simulink model "benchmarkss"  (Simulink 10.0)
settings: Solver=ode15s  StartTime=0.0  StopTime=200  FixedStep=0.01  RelTol=1e-5  AbsTol=1e-8
undefined symbols (not defined in the file or in its folder): carb1, carb2, carb3, carb4, carb5, carb6, carb7, KLa1, KLa2, KLa3, KLa4, KLa5, KLa6, KLa7, metal1, metal2, metal3, metal4, metal5, metal6, metal7, Qin0, Qintr, Qw
settings Model: Creator=ielulf  LastModifiedBy=xfal  ExtModeTrigMode=oneshot  ExtModeArmWhenConnect=off  ExtModeAutoUpdateStatusClock=off
settings SolverCC: AutoScaleAbsTol=off
settings DataIOCC: SignalLoggingSaveFormat=ModelDataLogs  SaveOutput=off  TimeSaveName=t  SignalLoggingName=sigsOut  OutputTimes=[0:(1):150]
settings OptimizationCC: BlockReduction=off  BooleanDataType=off  ExpressionDepthLimit=2147483647  InitFltsAndDblsToZero=on
settings DebuggingCC: AlgebraicLoopMsg=none  SaveWithParameterizedLinksMsg=none  SignalResolutionControl=TryResolveAllWithWarning  InheritedTsInSrcMsg=none  MultiTaskDSMMsg=warning  MultiTaskCondExecSysMsg=none  FcnCallInpInsideContextMsg=warning  UnconnectedOutputMsg=none  StateNameClashWarn=warning
settings HardwareCC: TargetUnknown=on
settings SFSimCC: SimUseLocalCustomCode=on  CustomCodeUndefinedFunction=FilterOut
settings RTWCC: TemplateMakefile=grt_unix.tmf  RTWUseLocalCustomCode=on
settings GRTTargetCC: TargetFcnLib=ansi_tfl_tmw.mat

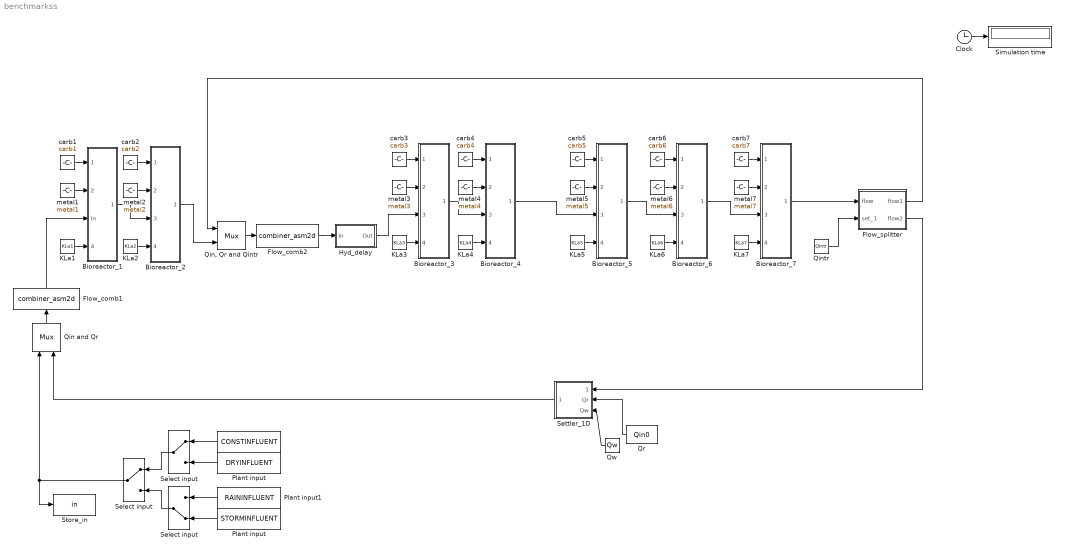
== system benchmarkss ==
  " " : FromWorkspace  VariableName=CONSTINFLUENT  OutputAfterFinalValue=Holding final value
  " Select input" : ManualSwitch
  Bioreactor_1 : Subsystem
  Bioreactor_2 : Subsystem
  Bioreactor_3 : Subsystem
  Bioreactor_4 : Subsystem
  Bioreactor_5 : Subsystem
  Bioreactor_6 : Subsystem
  Bioreactor_7 : Subsystem
  Clock : Clock
  Flow_comb1 : S-Function  FunctionName=combiner_asm2d  SFunctionDeploymentMode=off  EnableBusSupport=off
  Flow_comb2 : S-Function  FunctionName=combiner_asm2d  SFunctionDeploymentMode=off  EnableBusSupport=off
  Flow_splitter : Subsystem
  Hyd_delay : Subsystem
  KLa1 : Constant  Value=KLa1
  KLa2 : Constant  Value=KLa2
  KLa3 : Constant  Value=KLa3
  KLa4 : Constant  Value=KLa4
  KLa5 : Constant  Value=KLa5
  KLa6 : Constant  Value=KLa6
  KLa7 : Constant  Value=KLa7
  Plant input : FromWorkspace  VariableName=DRYINFLUENT  OutputAfterFinalValue=Holding final value
  "Plant input " : FromWorkspace  VariableName=STORMINFLUENT  OutputAfterFinalValue=Holding final value
  Plant input1 : FromWorkspace  VariableName=RAININFLUENT  OutputAfterFinalValue=Holding final value
  Qin and Qr : Mux  Inputs=2
  "Qin, Qr and Qintr" : Mux  Inputs=2
  Qintr : Constant  Value=Qintr
  Qr : Constant  Value=Qin0
  Qw : Constant  Value=Qw
  Select input : ManualSwitch
  "Select input " : ManualSwitch  CurrentSetting=0
  Settler_1D : Subsystem
  Simulation time : Display
  Store_in : ToWorkspace  VariableName=in  SampleTime=-1
  carb1 : Constant  Value=carb1
  carb2 : Constant  Value=carb2
  carb3 : Constant  Value=carb3
  carb4 : Constant  Value=carb4
  carb5 : Constant  Value=carb5
  carb6 : Constant  Value=carb6
  carb7 : Constant  Value=carb7
  metal1 : Constant  Value=metal1
  metal2 : Constant  Value=metal2
  metal3 : Constant  Value=metal3
  metal4 : Constant  Value=metal4
  metal5 : Constant  Value=metal5
  metal6 : Constant  Value=metal6
  metal7 : Constant  Value=metal7
  wires:
  Clock/1 -> Simulation time/1
  carb1/1 -> Bioreactor_1/1(carb)
  KLa1/1 -> Bioreactor_1/4(KLa)
  metal1/1 -> Bioreactor_1/2(metal)
  Flow_comb1/1 -> Bioreactor_1/3(in)
  Qin and Qr/1 -> Flow_comb1/1
  Plant input/1 -> Select input/2
  " "/1 -> Select input/1
  Plant input1/1 -> "Select input "/1
  "Plant input "/1 -> "Select input "/2
  Select input/1 -> " Select input"/1
  "Select input "/1 -> " Select input"/2
  " Select input"/1 -> Store_in/1, Qin and Qr/1
  Settler_1D/1(output) -> Qin and Qr/2
  Qw/1 -> Settler_1D/3(Qw)
  Qr/1 -> Settler_1D/2(Qr)
  Flow_splitter/2(flow2) -> Settler_1D/1(feed)
  "Qin, Qr and Qintr"/1 -> Flow_comb2/1
  Flow_comb2/1 -> Hyd_delay/1(In)
  KLa2/1 -> Bioreactor_2/4(KLa2)
  carb2/1 -> Bioreactor_2/1(carb2)
  metal2/1 -> Bioreactor_2/2(metal2)
  Bioreactor_1/1(out) -> Bioreactor_2/3(in1)
  Bioreactor_2/1(out1) -> "Qin, Qr and Qintr"/2
  KLa3/1 -> Bioreactor_3/4(KLa3)
  carb3/1 -> Bioreactor_3/1(carb3)
  metal3/1 -> Bioreactor_3/2(metal3)
  Hyd_delay/1(Out) -> Bioreactor_3/3(in1)
  KLa4/1 -> Bioreactor_4/4(KLa4)
  carb4/1 -> Bioreactor_4/1(carb4)
  metal4/1 -> Bioreactor_4/2(metal4)
  Bioreactor_3/1(out1) -> Bioreactor_4/3(in1)
  KLa5/1 -> Bioreactor_5/4(KLa5)
  carb5/1 -> Bioreactor_5/1(carb5)
  metal5/1 -> Bioreactor_5/2(metal5)
  Bioreactor_4/1(out1) -> Bioreactor_5/3(in1)
  KLa6/1 -> Bioreactor_6/4(KLa6)
  carb6/1 -> Bioreactor_6/1(carb6)
  metal6/1 -> Bioreactor_6/2(metal6)
  Bioreactor_5/1(out1) -> Bioreactor_6/3(in1)
  KLa7/1 -> Bioreactor_7/4(KLa7)
  carb7/1 -> Bioreactor_7/1(carb7)
  metal7/1 -> Bioreactor_7/2(metal7)
  Bioreactor_6/1(out1) -> Bioreactor_7/3(in1)
  Qintr/1 -> Flow_splitter/2(set_1)
  Bioreactor_7/1(out1) -> Flow_splitter/1(flow)
  Flow_splitter/1(flow1) -> "Qin, Qr and Qintr"/1

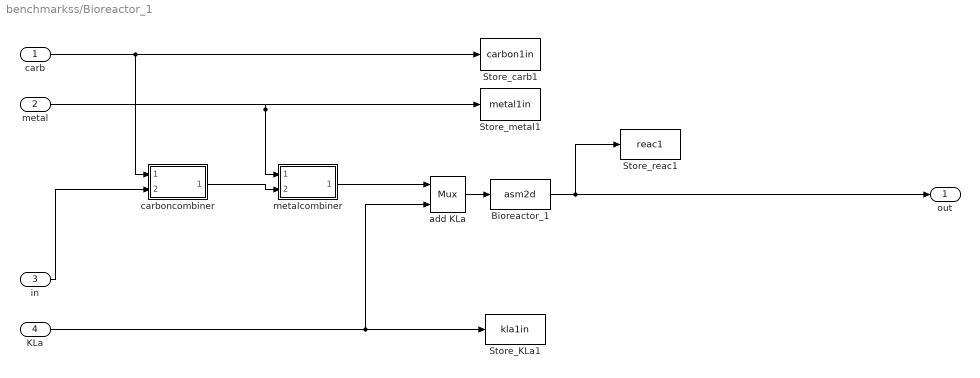
== system benchmarkss/Bioreactor_1 ==
  carb : Inport
  metal : Inport  Port=2
  in : Inport  Port=3
  KLa : Inport  Port=4
  Bioreactor_1 : S-Function  FunctionName=asm2d  Parameters=XINIT1,PAR1,VOL1,SOSAT1, DECAY, TEMPMODEL, ACTIVATE  SFunctionDeploymentMode=off  EnableBusSupport=off
  Store_KLa1 : ToWorkspace  VariableName=kla1in  SampleTime=-1
  Store_carb1 : ToWorkspace  VariableName=carbon1in  SampleTime=-1
  Store_metal1 : ToWorkspace  VariableName=metal1in  SampleTime=-1
  Store_reac1 : ToWorkspace  VariableName=reac1  SampleTime=-1
  add KLa : Mux  Inputs=2
  carboncombiner : Subsystem
  metalcombiner : Subsystem
  out : Outport
  wires:
  Bioreactor_1/1 -> Store_reac1/1, out/1
  in/1 -> carboncombiner/2(Input)
  KLa/1 -> Store_KLa1/1, add KLa/2
  carboncombiner/1(Output) -> metalcombiner/2(Input)
  metal/1 -> metalcombiner/1(C_flow), Store_metal1/1
  metalcombiner/1(Output) -> add KLa/1
  carb/1 -> carboncombiner/1(C_flow), Store_carb1/1
  add KLa/1 -> Bioreactor_1/1

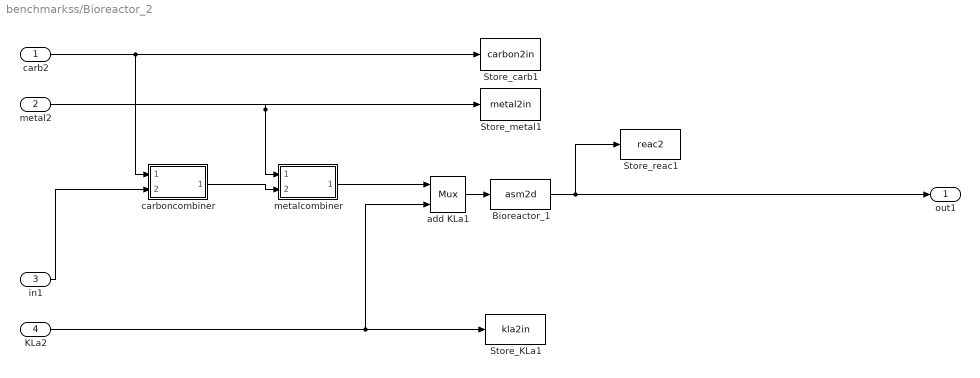
== system benchmarkss/Bioreactor_2 ==
  carb2 : Inport
  metal2 : Inport  Port=2
  in1 : Inport  Port=3
  KLa2 : Inport  Port=4
  Bioreactor_1 : S-Function  FunctionName=asm2d  Parameters=XINIT2,PAR2,VOL2,SOSAT2, DECAY, TEMPMODEL, ACTIVATE  SFunctionDeploymentMode=off  EnableBusSupport=off
  Store_KLa1 : ToWorkspace  VariableName=kla2in  SampleTime=-1
  Store_carb1 : ToWorkspace  VariableName=carbon2in  SampleTime=-1
  Store_metal1 : ToWorkspace  VariableName=metal2in  SampleTime=-1
  Store_reac1 : ToWorkspace  VariableName=reac2  SampleTime=-1
  add KLa1 : Mux  Inputs=2
  carboncombiner : Subsystem
  metalcombiner : Subsystem
  out1 : Outport
  wires:
  add KLa1/1 -> Bioreactor_1/1
  Bioreactor_1/1 -> Store_reac1/1, out1/1
  in1/1 -> carboncombiner/2(Input)
  KLa2/1 -> Store_KLa1/1, add KLa1/2
  carboncombiner/1(Output) -> metalcombiner/2(Input)
  metal2/1 -> metalcombiner/1(C_flow), Store_metal1/1
  metalcombiner/1(Output) -> add KLa1/1
  carb2/1 -> carboncombiner/1(C_flow), Store_carb1/1

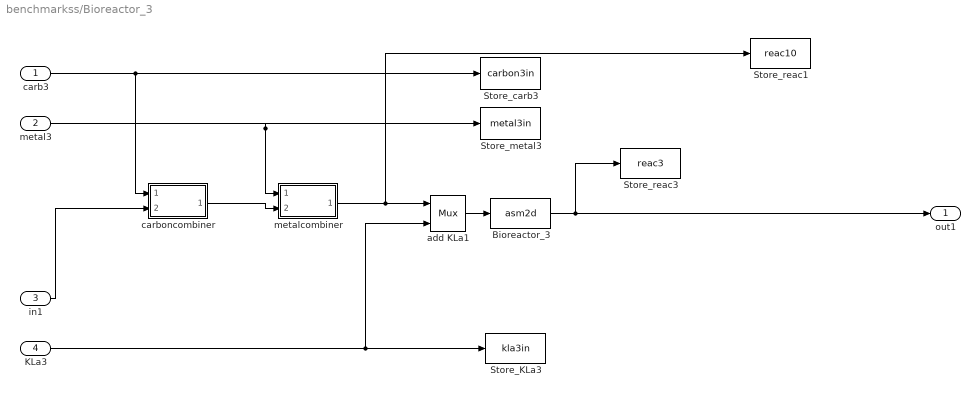
== system benchmarkss/Bioreactor_3 ==
  carb3 : Inport
  metal3 : Inport  Port=2
  in1 : Inport  Port=3
  KLa3 : Inport  Port=4
  Bioreactor_3 : S-Function  FunctionName=asm2d  Parameters=XINIT3,PAR3,VOL3,SOSAT3, DECAY,TEMPMODEL, ACTIVATE  SFunctionDeploymentMode=off  EnableBusSupport=off
  Store_KLa3 : ToWorkspace  VariableName=kla3in  SampleTime=-1
  Store_carb3 : ToWorkspace  VariableName=carbon3in  SampleTime=-1
  Store_metal3 : ToWorkspace  VariableName=metal3in  SampleTime=-1
  Store_reac1 : ToWorkspace  VariableName=reac10  SampleTime=-1
  Store_reac3 : ToWorkspace  VariableName=reac3  SampleTime=-1
  add KLa1 : Mux  Inputs=2
  carboncombiner : Subsystem
  metalcombiner : Subsystem
  out1 : Outport
  wires:
  add KLa1/1 -> Bioreactor_3/1
  Bioreactor_3/1 -> Store_reac3/1, out1/1
  in1/1 -> carboncombiner/2(Input)
  KLa3/1 -> Store_KLa3/1, add KLa1/2
  carboncombiner/1(Output) -> metalcombiner/2(Input)
  metal3/1 -> metalcombiner/1(C_flow), Store_metal3/1
  metalcombiner/1(Output) -> add KLa1/1, Store_reac1/1
  carb3/1 -> carboncombiner/1(C_flow), Store_carb3/1

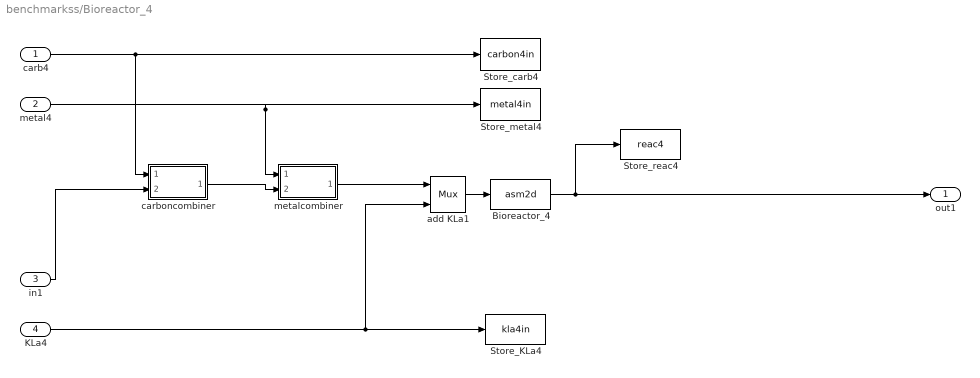
== system benchmarkss/Bioreactor_4 ==
  carb4 : Inport
  metal4 : Inport  Port=2
  in1 : Inport  Port=3
  KLa4 : Inport  Port=4
  Bioreactor_4 : S-Function  FunctionName=asm2d  Parameters=XINIT4,PAR4,VOL4,SOSAT4, DECAY,TEMPMODEL, ACTIVATE  SFunctionDeploymentMode=off  EnableBusSupport=off
  Store_KLa4 : ToWorkspace  VariableName=kla4in  SampleTime=-1
  Store_carb4 : ToWorkspace  VariableName=carbon4in  SampleTime=-1
  Store_metal4 : ToWorkspace  VariableName=metal4in  SampleTime=-1
  Store_reac4 : ToWorkspace  VariableName=reac4  SampleTime=-1
  add KLa1 : Mux  Inputs=2
  carboncombiner : Subsystem
  metalcombiner : Subsystem
  out1 : Outport
  wires:
  add KLa1/1 -> Bioreactor_4/1
  Bioreactor_4/1 -> Store_reac4/1, out1/1
  in1/1 -> carboncombiner/2(Input)
  KLa4/1 -> Store_KLa4/1, add KLa1/2
  carboncombiner/1(Output) -> metalcombiner/2(Input)
  metal4/1 -> metalcombiner/1(C_flow), Store_metal4/1
  metalcombiner/1(Output) -> add KLa1/1
  carb4/1 -> carboncombiner/1(C_flow), Store_carb4/1

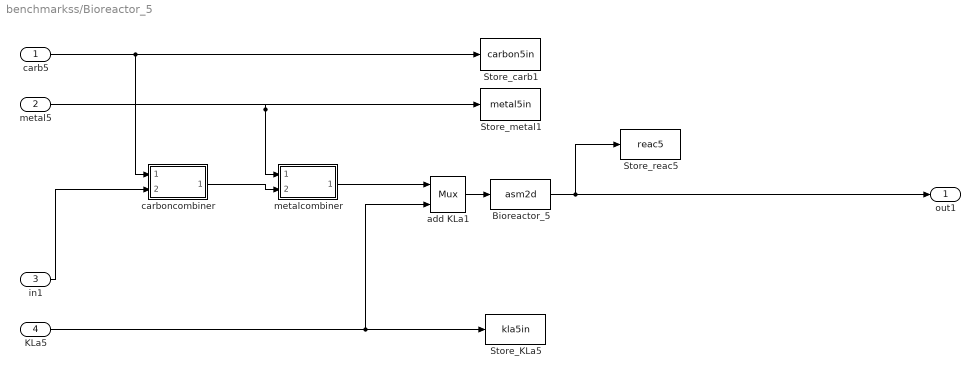
== system benchmarkss/Bioreactor_5 ==
  carb5 : Inport
  metal5 : Inport  Port=2
  in1 : Inport  Port=3
  KLa5 : Inport  Port=4
  Bioreactor_5 : S-Function  FunctionName=asm2d  Parameters=XINIT5,PAR5,VOL5,SOSAT5, DECAY, TEMPMODEL, ACTIVATE  SFunctionDeploymentMode=off  EnableBusSupport=off
  Store_KLa5 : ToWorkspace  VariableName=kla5in  SampleTime=-1
  Store_carb1 : ToWorkspace  VariableName=carbon5in  SampleTime=-1
  Store_metal1 : ToWorkspace  VariableName=metal5in  SampleTime=-1
  Store_reac5 : ToWorkspace  VariableName=reac5  SampleTime=-1
  add KLa1 : Mux  Inputs=2
  carboncombiner : Subsystem
  metalcombiner : Subsystem
  out1 : Outport
  wires:
  add KLa1/1 -> Bioreactor_5/1
  Bioreactor_5/1 -> Store_reac5/1, out1/1
  in1/1 -> carboncombiner/2(Input)
  KLa5/1 -> Store_KLa5/1, add KLa1/2
  carboncombiner/1(Output) -> metalcombiner/2(Input)
  metal5/1 -> metalcombiner/1(C_flow), Store_metal1/1
  metalcombiner/1(Output) -> add KLa1/1
  carb5/1 -> carboncombiner/1(C_flow), Store_carb1/1

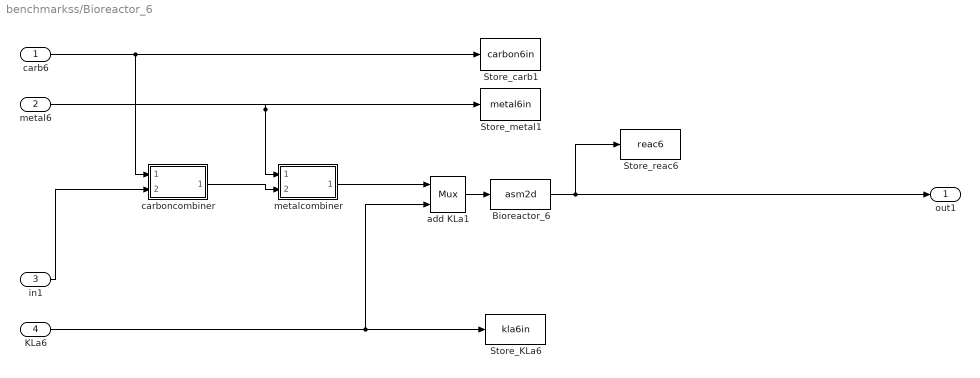
== system benchmarkss/Bioreactor_6 ==
  carb6 : Inport
  metal6 : Inport  Port=2
  in1 : Inport  Port=3
  KLa6 : Inport  Port=4
  Bioreactor_6 : S-Function  FunctionName=asm2d  Parameters=XINIT6,PAR6,VOL6,SOSAT6, DECAY, TEMPMODEL, ACTIVATE  SFunctionDeploymentMode=off  EnableBusSupport=off
  Store_KLa6 : ToWorkspace  VariableName=kla6in  SampleTime=-1
  Store_carb1 : ToWorkspace  VariableName=carbon6in  SampleTime=-1
  Store_metal1 : ToWorkspace  VariableName=metal6in  SampleTime=-1
  Store_reac6 : ToWorkspace  VariableName=reac6  SampleTime=-1
  add KLa1 : Mux  Inputs=2
  carboncombiner : Subsystem
  metalcombiner : Subsystem
  out1 : Outport
  wires:
  add KLa1/1 -> Bioreactor_6/1
  Bioreactor_6/1 -> Store_reac6/1, out1/1
  in1/1 -> carboncombiner/2(Input)
  KLa6/1 -> Store_KLa6/1, add KLa1/2
  carboncombiner/1(Output) -> metalcombiner/2(Input)
  metal6/1 -> metalcombiner/1(C_flow), Store_metal1/1
  metalcombiner/1(Output) -> add KLa1/1
  carb6/1 -> carboncombiner/1(C_flow), Store_carb1/1

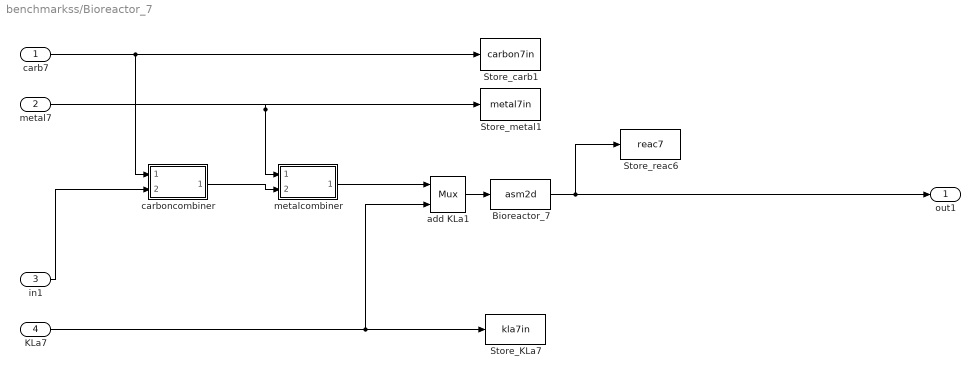
== system benchmarkss/Bioreactor_7 ==
  carb7 : Inport
  metal7 : Inport  Port=2
  in1 : Inport  Port=3
  KLa7 : Inport  Port=4
  Bioreactor_7 : S-Function  FunctionName=asm2d  Parameters=XINIT7,PAR7,VOL7,SOSAT7, DECAY, TEMPMODEL, ACTIVATE  SFunctionDeploymentMode=off  EnableBusSupport=off
  Store_KLa7 : ToWorkspace  VariableName=kla7in  SampleTime=-1
  Store_carb1 : ToWorkspace  VariableName=carbon7in  SampleTime=-1
  Store_metal1 : ToWorkspace  VariableName=metal7in  SampleTime=-1
  Store_reac6 : ToWorkspace  VariableName=reac7  SampleTime=-1
  add KLa1 : Mux  Inputs=2
  carboncombiner : Subsystem
  metalcombiner : Subsystem
  out1 : Outport
  wires:
  add KLa1/1 -> Bioreactor_7/1
  Bioreactor_7/1 -> Store_reac6/1, out1/1
  in1/1 -> carboncombiner/2(Input)
  KLa7/1 -> Store_KLa7/1, add KLa1/2
  carboncombiner/1(Output) -> metalcombiner/2(Input)
  metal7/1 -> metalcombiner/1(C_flow), Store_metal1/1
  metalcombiner/1(Output) -> add KLa1/1
  carb7/1 -> carboncombiner/1(C_flow), Store_carb1/1

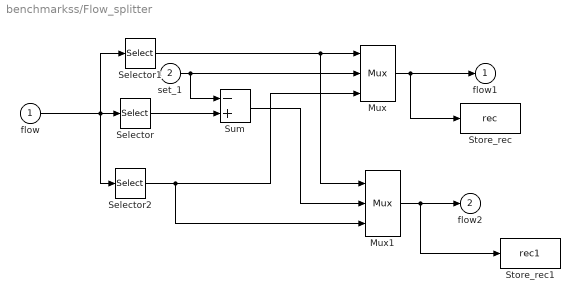
== system benchmarkss/Flow_splitter ==
  flow : Inport
  set_1 : Inport  Port=2
  Mux : Mux  Inputs=3
  Mux1 : Mux  Inputs=3
  Selector : Selector  InputPortWidth=26  IndexOptions=Index vector (dialog)  Indices=[20]  OutputSizes=1
  Selector1 : Selector  InputPortWidth=26  IndexOptions=Index vector (dialog)  Indices=[1 2 3 4 5 6 7 8 9 10 11 12 13 14 15 16 17 18 19 ]  OutputSizes=1
  Selector2 : Selector  InputPortWidth=26  IndexOptions=Index vector (dialog)  Indices=[21 22 23 24 25 26]  OutputSizes=1
  Store_rec : ToWorkspace  VariableName=rec  SampleTime=-1
  Store_rec1 : ToWorkspace  VariableName=rec1  SampleTime=-1
  Sum : Sum  Inputs=-+  SaturateOnIntegerOverflow=on  InputSameDT=on  OutDataTypeStr=Inherit: Same as first input
  flow1 : Outport
  flow2 : Outport  Port=2
  wires:
  flow/1 -> Selector1/1, Selector/1, Selector2/1
  Mux/1 -> flow1/1, Store_rec/1
  Mux1/1 -> flow2/1, Store_rec1/1
  set_1/1 -> Mux/2, Sum/1
  Selector/1 -> Sum/2
  Sum/1 -> Mux1/2
  Selector1/1 -> Mux/1, Mux1/1
  Selector2/1 -> Mux/3, Mux1/3

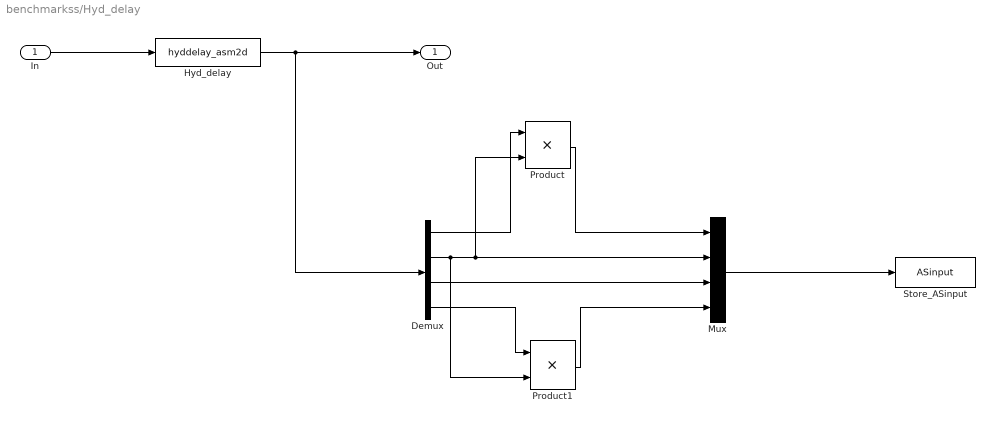
== system benchmarkss/Hyd_delay ==
  In : Inport
  Demux : Demux  Outputs=[19,1,1,5]
  Hyd_delay : S-Function  FunctionName=hyddelay_asm2d  Parameters=XINITDELAY,PAR1, T  SFunctionDeploymentMode=off  EnableBusSupport=off
  Mux : Mux
  Product : Product  SaturateOnIntegerOverflow=on  OutDataTypeStr=Inherit: Same as first input
  Product1 : Product  SaturateOnIntegerOverflow=on  OutDataTypeStr=Inherit: Same as first input
  Store_ASinput : ToWorkspace  VariableName=ASinput  SampleTime=-1
  Out : Outport
  wires:
  In/1 -> Hyd_delay/1
  Hyd_delay/1 -> Out/1, Demux/1
  Demux/1 -> Product/1
  Product/1 -> Mux/1
  Mux/1 -> Store_ASinput/1
  Demux/4 -> Product1/1
  Product1/1 -> Mux/4
  Demux/3 -> Mux/3
  Demux/2 -> Product1/2, Mux/2, Product/2

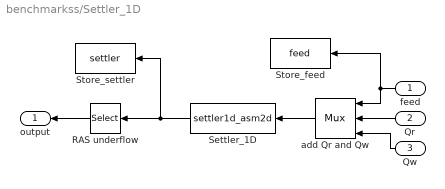
== system benchmarkss/Settler_1D ==
  feed : Inport
  Qr : Inport  Port=2
  Qw : Inport  Port=3
  RAS underflow : Selector  InputPortWidth=316  IndexOptions=Index vector (dialog)  Indices=[1 2 3 4 5 6 7 8 9 10 11 12 13 14 15 16 17 18 19 20 21 22 23 24 25 26]  OutputSizes=1
  Settler_1D : S-Function  FunctionName=settler1d_asm2d  Parameters=SETTLERINIT2D,SETTLERPAR2D,DIM2D,LAYER2D,ASM2DPAR, DECAY, SETTLER, TEMPMODEL  SFunctionDeploymentMode=off  EnableBusSupport=off
  Store_feed : ToWorkspace  VariableName=feed  SampleTime=-1
  Store_settler : ToWorkspace  VariableName=settler  SampleTime=-1
  add Qr and Qw : Mux  Inputs=3
  output : Outport
  wires:
  add Qr and Qw/1 -> Settler_1D/1
  Qr/1 -> add Qr and Qw/2
  Qw/1 -> add Qr and Qw/3
  feed/1 -> add Qr and Qw/1, Store_feed/1
  RAS underflow/1 -> output/1
  Settler_1D/1 -> RAS underflow/1, Store_settler/1

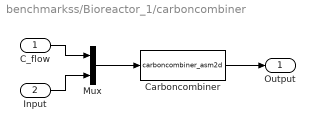
== system benchmarkss/Bioreactor_1/carboncombiner ==
  C_flow : Inport
  Input : Inport  Port=2
  Carboncombiner : S-Function  FunctionName=carboncombiner_asm2d  Parameters=CARBONSOURCECONC  SFunctionDeploymentMode=off  EnableBusSupport=off
  Mux : Mux  Inputs=2
  Output : Outport
  wires:
  C_flow/1 -> Mux/1
  Mux/1 -> Carboncombiner/1
  Carboncombiner/1 -> Output/1
  Input/1 -> Mux/2

== system benchmarkss/Bioreactor_1/metalcombiner ==
  C_flow : Inport
  Input : Inport  Port=2
  Carboncombiner : S-Function  FunctionName=metalcombiner_asm2d  Parameters=METALSOURCECONC  SFunctionDeploymentMode=off  EnableBusSupport=off
  Mux : Mux  Inputs=2
  Output : Outport
  wires:
  C_flow/1 -> Mux/1
  Mux/1 -> Carboncombiner/1
  Carboncombiner/1 -> Output/1
  Input/1 -> Mux/2

== system benchmarkss/Bioreactor_2/carboncombiner ==
  C_flow : Inport
  Input : Inport  Port=2
  Carboncombiner : S-Function  FunctionName=carboncombiner_asm2d  Parameters=CARBONSOURCECONC  SFunctionDeploymentMode=off  EnableBusSupport=off
  Mux : Mux  Inputs=2
  Output : Outport
  wires:
  C_flow/1 -> Mux/1
  Mux/1 -> Carboncombiner/1
  Carboncombiner/1 -> Output/1
  Input/1 -> Mux/2

== system benchmarkss/Bioreactor_2/metalcombiner ==
  C_flow : Inport
  Input : Inport  Port=2
  Carboncombiner : S-Function  FunctionName=metalcombiner_asm2d  Parameters=METALSOURCECONC  SFunctionDeploymentMode=off  EnableBusSupport=off
  Mux : Mux  Inputs=2
  Output : Outport
  wires:
  C_flow/1 -> Mux/1
  Mux/1 -> Carboncombiner/1
  Carboncombiner/1 -> Output/1
  Input/1 -> Mux/2

== system benchmarkss/Bioreactor_3/carboncombiner ==
  C_flow : Inport
  Input : Inport  Port=2
  Carboncombiner : S-Function  FunctionName=carboncombiner_asm2d  Parameters=CARBONSOURCECONC  SFunctionDeploymentMode=off  EnableBusSupport=off
  Mux : Mux  Inputs=2
  Output : Outport
  wires:
  C_flow/1 -> Mux/1
  Mux/1 -> Carboncombiner/1
  Carboncombiner/1 -> Output/1
  Input/1 -> Mux/2

== system benchmarkss/Bioreactor_3/metalcombiner ==
  C_flow : Inport
  Input : Inport  Port=2
  Carboncombiner : S-Function  FunctionName=metalcombiner_asm2d  Parameters=METALSOURCECONC  SFunctionDeploymentMode=off  EnableBusSupport=off
  Mux : Mux  Inputs=2
  Output : Outport
  wires:
  C_flow/1 -> Mux/1
  Mux/1 -> Carboncombiner/1
  Carboncombiner/1 -> Output/1
  Input/1 -> Mux/2

== system benchmarkss/Bioreactor_4/carboncombiner ==
  C_flow : Inport
  Input : Inport  Port=2
  Carboncombiner : S-Function  FunctionName=carboncombiner_asm2d  Parameters=CARBONSOURCECONC  SFunctionDeploymentMode=off  EnableBusSupport=off
  Mux : Mux  Inputs=2
  Output : Outport
  wires:
  C_flow/1 -> Mux/1
  Mux/1 -> Carboncombiner/1
  Carboncombiner/1 -> Output/1
  Input/1 -> Mux/2

== system benchmarkss/Bioreactor_4/metalcombiner ==
  C_flow : Inport
  Input : Inport  Port=2
  Carboncombiner : S-Function  FunctionName=metalcombiner_asm2d  Parameters=METALSOURCECONC  SFunctionDeploymentMode=off  EnableBusSupport=off
  Mux : Mux  Inputs=2
  Output : Outport
  wires:
  C_flow/1 -> Mux/1
  Mux/1 -> Carboncombiner/1
  Carboncombiner/1 -> Output/1
  Input/1 -> Mux/2

== system benchmarkss/Bioreactor_5/carboncombiner ==
  C_flow : Inport
  Input : Inport  Port=2
  Carboncombiner : S-Function  FunctionName=carboncombiner_asm2d  Parameters=CARBONSOURCECONC  SFunctionDeploymentMode=off  EnableBusSupport=off
  Mux : Mux  Inputs=2
  Output : Outport
  wires:
  C_flow/1 -> Mux/1
  Mux/1 -> Carboncombiner/1
  Carboncombiner/1 -> Output/1
  Input/1 -> Mux/2

== system benchmarkss/Bioreactor_5/metalcombiner ==
  C_flow : Inport
  Input : Inport  Port=2
  Carboncombiner : S-Function  FunctionName=metalcombiner_asm2d  Parameters=METALSOURCECONC  SFunctionDeploymentMode=off  EnableBusSupport=off
  Mux : Mux  Inputs=2
  Output : Outport
  wires:
  C_flow/1 -> Mux/1
  Mux/1 -> Carboncombiner/1
  Carboncombiner/1 -> Output/1
  Input/1 -> Mux/2

== system benchmarkss/Bioreactor_6/carboncombiner ==
  C_flow : Inport
  Input : Inport  Port=2
  Carboncombiner : S-Function  FunctionName=carboncombiner_asm2d  Parameters=CARBONSOURCECONC  SFunctionDeploymentMode=off  EnableBusSupport=off
  Mux : Mux  Inputs=2
  Output : Outport
  wires:
  C_flow/1 -> Mux/1
  Mux/1 -> Carboncombiner/1
  Carboncombiner/1 -> Output/1
  Input/1 -> Mux/2

== system benchmarkss/Bioreactor_6/metalcombiner ==
  C_flow : Inport
  Input : Inport  Port=2
  Carboncombiner : S-Function  FunctionName=metalcombiner_asm2d  Parameters=METALSOURCECONC  SFunctionDeploymentMode=off  EnableBusSupport=off
  Mux : Mux  Inputs=2
  Output : Outport
  wires:
  C_flow/1 -> Mux/1
  Mux/1 -> Carboncombiner/1
  Carboncombiner/1 -> Output/1
  Input/1 -> Mux/2

== system benchmarkss/Bioreactor_7/carboncombiner ==
  C_flow : Inport
  Input : Inport  Port=2
  Carboncombiner : S-Function  FunctionName=carboncombiner_asm2d  Parameters=CARBONSOURCECONC  SFunctionDeploymentMode=off  EnableBusSupport=off
  Mux : Mux  Inputs=2
  Output : Outport
  wires:
  C_flow/1 -> Mux/1
  Mux/1 -> Carboncombiner/1
  Carboncombiner/1 -> Output/1
  Input/1 -> Mux/2

== system benchmarkss/Bioreactor_7/metalcombiner ==
  C_flow : Inport
  Input : Inport  Port=2
  Carboncombiner : S-Function  FunctionName=metalcombiner_asm2d  Parameters=METALSOURCECONC  SFunctionDeploymentMode=off  EnableBusSupport=off
  Mux : Mux  Inputs=2
  Output : Outport
  wires:
  C_flow/1 -> Mux/1
  Mux/1 -> Carboncombiner/1
  Carboncombiner/1 -> Output/1
  Input/1 -> Mux/2
